simulink model "FuelT_VD"  (R2016b)
settings: configuration reference "CodeGenConfigSet" (kept outside this file)
values from neighbouring files (symbols this model uses):
  FuelT_facSerPT1T_C = Calibration.Parameter    [init_FuelT_VD.m]    (also in init_FuelT_VD_SIL.m = Simulink.Parameter)
  FuelT_RmpSlpNeg_C = Calibration.Parameter    [init_FuelT_VD.m]    (also in init_FuelT_VD_SIL.m = Simulink.Parameter)
  FuelT_RmpSlpPos_C = Calibration.Parameter    [init_FuelT_VD.m]    (also in init_FuelT_VD_SIL.m = Simulink.Parameter)
  FuelT_swtTempSel_C = Calibration.Parameter    [init_FuelT_VD.m]    (also in init_FuelT_VD_SIL.m = Simulink.Parameter)
  FuelT_tDflFlSys_C = Calibration.Parameter    [init_FuelT_VD.m]    (also in init_FuelT_VD_SIL.m = Simulink.Parameter)
  FuelT_tTransStgDfl_C = Calibration.Parameter    [init_FuelT_VD.m]    (also in init_FuelT_VD_SIL.m = Simulink.Parameter)
  SigTst_swtFuelT_C = Calibration.Parameter    [init_FuelT_VD.m]    (also in init_FuelT_VD_SIL.m = Simulink.Parameter)
  SigTst_tFuelT_C = Calibration.Parameter    [init_FuelT_VD.m]    (also in init_FuelT_VD_SIL.m = Simulink.Parameter)
undefined symbols (not defined in the file or in its folder): CEngDst_switch_conv, FuelT_VD_DT, Switch_conv
libraries: CXLib x8
settings Model: Creator=Wollf  LastModifiedBy=dulinggang
settings ConfigSetRef: SourceLocation=Base Workspace

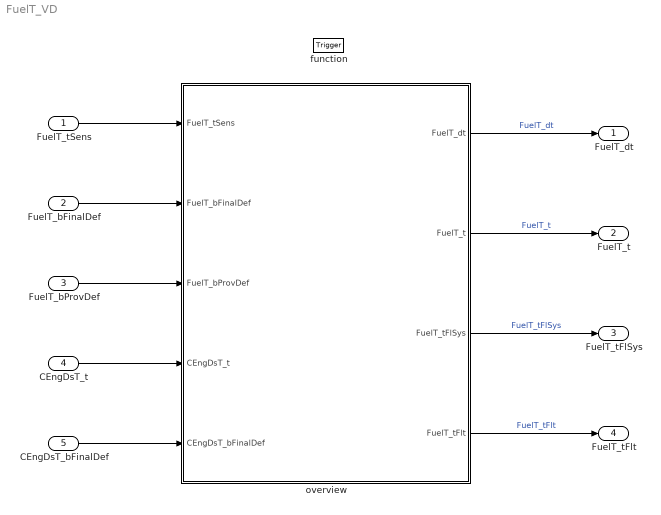
== system FuelT_VD ==
  FuelT_tSens : Inport  Tag=deg  Description=Sensed fuel temperature  OutMin=-50  OutMax=150  OutDataTypeStr=Temp_deg
  FuelT_bFinalDef : Inport  Description=Status sensor of the fuel temperature finally defect  Port=2  OutMin=0  OutMax=1  OutDataTypeStr=boolean
  FuelT_bProvDef : Inport  Description=Status sensor of the fuel temperature temporary defect  Port=3  OutMin=0  OutMax=1  OutDataTypeStr=boolean
  CEngDsT_t : Inport  Tag=deg  Description=engine coolant temperature after filter  Port=4  OutMin=-200  OutMax=200  OutDataTypeStr=Temp_deg
  CEngDsT_bFinalDef : Inport  Description=Status Sensor of the coolant temperature finally defect  Port=5  OutMin=0  OutMax=1  OutDataTypeStr=boolean
  function : TriggerPort  TriggerType=function-call  VariantControl=Variant
  overview : Subsystem
  FuelT_dt : Outport  Tag=deg/s  Description=temperature change rate  OutMin=-200  OutMax=200  OutDataTypeStr=Temp_deg_s
  FuelT_t : Outport  Tag=deg  Description=Temperature of fuel  Port=2  OutMin=-50  OutMax=150  OutDataTypeStr=Temp_deg
  FuelT_tFlSys : Outport  Tag=deg  Description=Fuel system temperature  Port=3  OutMin=-50  OutMax=200  OutDataTypeStr=Temp_deg
  FuelT_tFlt : Outport  Tag=deg  Description=fuel temperature after filter  Port=4  OutMin=-50  OutMax=150  OutDataTypeStr=Temp_deg
  wires:
  FuelT_tSens/1 -> overview/1(FuelT_tSens)
  FuelT_bFinalDef/1 -> overview/2(FuelT_bFinalDef)
  FuelT_bProvDef/1 -> overview/3(FuelT_bProvDef)
  CEngDsT_t/1 -> overview/4(CEngDsT_t)
  CEngDsT_bFinalDef/1 -> overview/5(CEngDsT_bFinalDef)
  overview/1(FuelT_dt) -> FuelT_dt/1  "FuelT_dt"
  overview/2(FuelT_t) -> FuelT_t/1  "FuelT_t"
  overview/3(FuelT_tFlSys) -> FuelT_tFlSys/1  "FuelT_tFlSys"
  overview/4(FuelT_tFlt) -> FuelT_tFlt/1  "FuelT_tFlt"

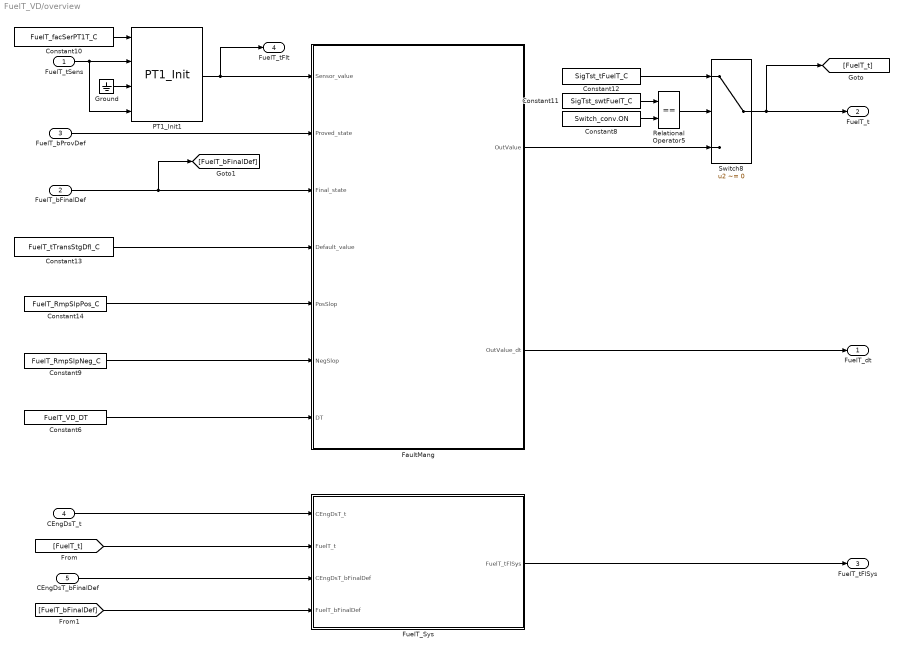
== system FuelT_VD/overview ==
  FuelT_tSens : Inport  Tag=deg  Description=Sensed fuel temperature  OutMin=-50  OutMax=150  OutDataTypeStr=Temp_deg
  FuelT_bFinalDef : Inport  Description=Status sensor of the fuel temperature finally defect  Port=2  OutMin=0  OutMax=1  OutDataTypeStr=boolean
  FuelT_bProvDef : Inport  Description=Status sensor of the fuel temperature temporary defect  Port=3  OutMin=0  OutMax=1  OutDataTypeStr=boolean
  CEngDsT_t : Inport  Tag=deg  Description=engine coolant temperature after filter  Port=4  OutMin=-200  OutMax=200  OutDataTypeStr=Temp_deg
  CEngDsT_bFinalDef : Inport  Description=Status Sensor of the coolant temperature finally defect  Port=5  OutMin=0  OutMax=1  OutDataTypeStr=boolean
  Constant10 : Constant  Value=FuelT_facSerPT1T_C  SampleTime=-1
  Constant11 : Constant  Value=SigTst_swtFuelT_C  SampleTime=-1
  Constant12 : Constant  Value=SigTst_tFuelT_C  SampleTime=-1
  Constant13 : Constant  Value=FuelT_tTransStgDfl_C  SampleTime=-1
  Constant14 : Constant  Value=FuelT_RmpSlpPos_C  SampleTime=-1
  Constant6 : Constant  Value=FuelT_VD_DT  OutDataTypeStr=int16  SampleTime=-1
  Constant8 : Constant  Value=Switch_conv.ON  OutDataTypeStr=Inherit: Inherit via back propagation
  Constant9 : Constant  Value=FuelT_RmpSlpNeg_C  SampleTime=-1
  FaultMang : Subsystem
  FuelT_Sys : Subsystem
  Ground : Ground
  PT1_Init1 : CXLib/PT1_Init
  Relational Operator5 : RelationalOperator  Operator===  OutDataTypeStr=boolean  RndMeth=Simplest  InputSameDT=on
  Switch8 : Switch  Criteria=u2 ~= 0  Threshold=CEngDst_switch_conv.OFF  InputSameDT=on
  FuelT_dt : Outport  Tag=deg/s  Description=temperature change rate  OutMin=-200  OutMax=200  OutDataTypeStr=Temp_deg_s
  FuelT_t : Outport  Tag=deg  Description=Temperature of fuel  Port=2  OutMin=-50  OutMax=150  OutDataTypeStr=Temp_deg
  FuelT_tFlSys : Outport  Tag=deg  Description=Fuel system temperature  Port=3  OutMin=-50  OutMax=200  OutDataTypeStr=Temp_deg
  FuelT_tFlt : Outport  Tag=deg  Description=fuel temperature after filter  Port=4  OutMin=-50  OutMax=150  OutDataTypeStr=Temp_deg
  wires:
  FuelT_bFinalDef/1 -> FaultMang/3(Final_state), [FuelT_bFinalDef]
  PT1_Init1/1 -> FuelT_tFlt/1, FaultMang/1(Sensor_value)
  Constant13/1 -> FaultMang/4(Default_value)
  Relational Operator5/1 -> Switch8/2
  Constant8/1 -> Relational Operator5/2
  Ground/1 -> PT1_Init1/3
  Constant14/1 -> FaultMang/5(PosSlop)
  FuelT_Sys/1(FuelT_tFlSys) -> FuelT_tFlSys/1
  Constant12/1 -> Switch8/1
  FuelT_tSens/1 -> PT1_Init1/4, PT1_Init1/2
  Constant10/1 -> PT1_Init1/1
  Constant11/1 -> Relational Operator5/1
  Switch8/1 -> FuelT_t/1, [FuelT_t]
  Constant6/1 -> FaultMang/7(DT)
  Constant9/1 -> FaultMang/6(NegSlop)
  [FuelT_t] -> FuelT_Sys/2(FuelT_t)
  [FuelT_bFinalDef] -> FuelT_Sys/4(FuelT_bFinalDef)
  CEngDsT_bFinalDef/1 -> FuelT_Sys/3(CEngDsT_bFinalDef)
  FuelT_bProvDef/1 -> FaultMang/2(Proved_state)
  CEngDsT_t/1 -> FuelT_Sys/1(CEngDsT_t)
  FaultMang/1(OutValue) -> Switch8/3
  FaultMang/2(OutValue_dt) -> FuelT_dt/1

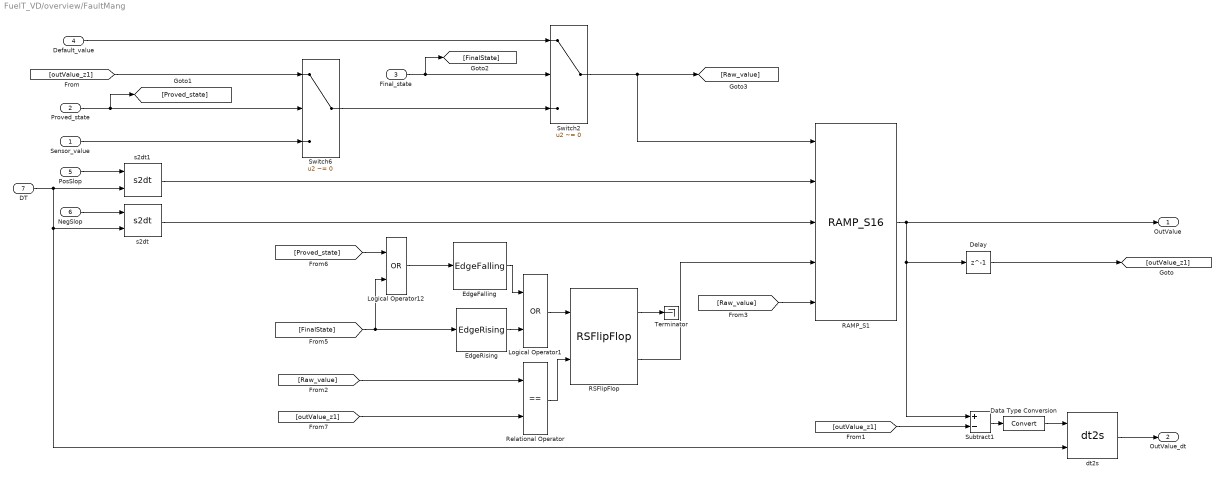
== system FuelT_VD/overview/FaultMang ==
  Sensor_value : Inport
  Proved_state : Inport  Port=2
  Final_state : Inport  Port=3
  Default_value : Inport  Port=4
  PosSlop : Inport  Port=5
  NegSlop : Inport  Port=6
  DT : Inport  Port=7
  Data Type Conversion : DataTypeConversion
  Delay : Delay  DialogController=Simulink.DDGSource  DelayLength=1  InitialCondition=0
  EdgeFalling : CXLib/EdgeFalling
  EdgeRising : CXLib/EdgeRising
  Logical Operator1 : Logic  Operator=OR  OutDataTypeStr=boolean
  Logical Operator12 : Logic  Operator=OR  OutDataTypeStr=boolean
  RAMP_S1 : CXLib/RAMP_S16
  RSFlipFlop : CXLib/RSFlipFlop
  Relational Operator : RelationalOperator  Operator===  OutDataTypeStr=boolean  RndMeth=Simplest
  Subtract1 : Sum  Inputs=+-
  Switch2 : Switch  Criteria=u2 ~= 0  InputSameDT=on
  Switch6 : Switch  Criteria=u2 ~= 0  InputSameDT=on
  Terminator : Terminator
  dt2s : CXLib/dt2s
  s2dt : CXLib/s2dt
  s2dt1 : CXLib/s2dt
  OutValue : Outport
  OutValue_dt : Outport  Port=2
  wires:
  Switch2/1 -> RAMP_S1/1, [Raw_value]
  Logical Operator12/1 -> EdgeFalling/1
  RSFlipFlop/1 -> Terminator/1
  Relational Operator/1 -> RSFlipFlop/2
  RAMP_S1/1 -> Subtract1/1, Delay/1, OutValue/1
  Default_value/1 -> Switch2/1
  Switch6/1 -> Switch2/3
  Delay/1 -> [outValue_z1]
  [outValue_z1] -> Switch6/1
  Final_state/1 -> [FinalState], Switch2/2
  DT/1 -> dt2s/2, s2dt/2, s2dt1/2
  Proved_state/1 -> Switch6/2, [Proved_state]
  [FinalState] -> Logical Operator12/2, EdgeRising/1
  [Proved_state] -> Logical Operator12/1
  Sensor_value/1 -> Switch6/3
  [Raw_value] -> RAMP_S1/5
  [outValue_z1] -> Relational Operator/2
  Logical Operator1/1 -> RSFlipFlop/1
  EdgeRising/1 -> Logical Operator1/2
  EdgeFalling/1 -> Logical Operator1/1
  RSFlipFlop/2 -> RAMP_S1/4
  dt2s/1 -> OutValue_dt/1
  [Raw_value] -> Relational Operator/1
  Subtract1/1 -> Data Type Conversion/1
  Data Type Conversion/1 -> dt2s/1
  [outValue_z1] -> Subtract1/2
  NegSlop/1 -> s2dt/1
  s2dt/1 -> RAMP_S1/3
  PosSlop/1 -> s2dt1/1
  s2dt1/1 -> RAMP_S1/2

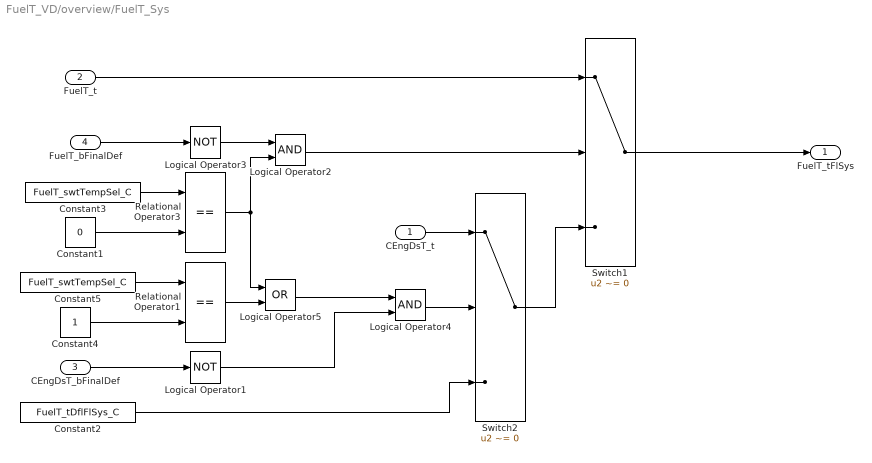
== system FuelT_VD/overview/FuelT_Sys ==
  CEngDsT_t : Inport  Tag=deg  Description=engine coolant temperature after filter  OutMin=-200  OutMax=200  OutDataTypeStr=Temp_deg
  FuelT_t : Inport  Tag=deg  Description=engine coolant temperature after filter  Port=2  OutMin=-200  OutMax=200  OutDataTypeStr=Temp_deg
  CEngDsT_bFinalDef : Inport  Description=Status Sensor of the coolant temperature finally defect  Port=3  OutMin=0  OutMax=1  OutDataTypeStr=boolean
  FuelT_bFinalDef : Inport  Description=Status sensor of the fuel temperature finally defect  Port=4  OutMin=0  OutMax=1  OutDataTypeStr=boolean
  Constant1 : Constant  Value=0
  Constant2 : Constant  Value=FuelT_tDflFlSys_C  SampleTime=-1
  Constant3 : Constant  Value=FuelT_swtTempSel_C  SampleTime=-1
  Constant4 : Constant
  Constant5 : Constant  Value=FuelT_swtTempSel_C  SampleTime=-1
  Logical Operator1 : Logic  Operator=NOT  AllPortsSameDT=off  OutDataTypeStr=boolean
  Logical Operator2 : Logic  AllPortsSameDT=off  OutDataTypeStr=boolean
  Logical Operator3 : Logic  Operator=NOT  AllPortsSameDT=off  OutDataTypeStr=boolean
  Logical Operator4 : Logic  AllPortsSameDT=off  OutDataTypeStr=boolean
  Logical Operator5 : Logic  Operator=OR  AllPortsSameDT=off  OutDataTypeStr=boolean
  Relational Operator1 : RelationalOperator  Operator===  OutDataTypeStr=boolean  RndMeth=Simplest
  Relational Operator3 : RelationalOperator  Operator===  OutDataTypeStr=boolean  RndMeth=Simplest
  Switch1 : Switch  Criteria=u2 ~= 0  InputSameDT=on
  Switch2 : Switch  Criteria=u2 ~= 0  InputSameDT=on
  FuelT_tFlSys : Outport  Tag=deg  Description=Fuel system temperature  OutMin=-50  OutMax=200  OutDataTypeStr=Temp_deg
  wires:
  FuelT_bFinalDef/1 -> Logical Operator3/1
  Logical Operator3/1 -> Logical Operator2/1
  FuelT_t/1 -> Switch1/1
  Logical Operator2/1 -> Switch1/2
  Switch2/1 -> Switch1/3
  CEngDsT_t/1 -> Switch2/1
  CEngDsT_bFinalDef/1 -> Logical Operator1/1
  Constant2/1 -> Switch2/3
  Switch1/1 -> FuelT_tFlSys/1
  Constant3/1 -> Relational Operator3/1
  Constant1/1 -> Relational Operator3/2
  Relational Operator3/1 -> Logical Operator5/1, Logical Operator2/2
  Logical Operator1/1 -> Logical Operator4/2
  Logical Operator4/1 -> Switch2/2
  Constant5/1 -> Relational Operator1/1
  Constant4/1 -> Relational Operator1/2
  Relational Operator1/1 -> Logical Operator5/2
  Logical Operator5/1 -> Logical Operator4/1
